simulink subsystem "Sensores"  (R2022b)
settings: Solver=VariableStepAuto  StartTime=0.0  StopTime=10.0  RelTol=1e-3
libraries: arduinolib x2
settings Model: Creator=mmgac  LastModifiedBy=mmgac

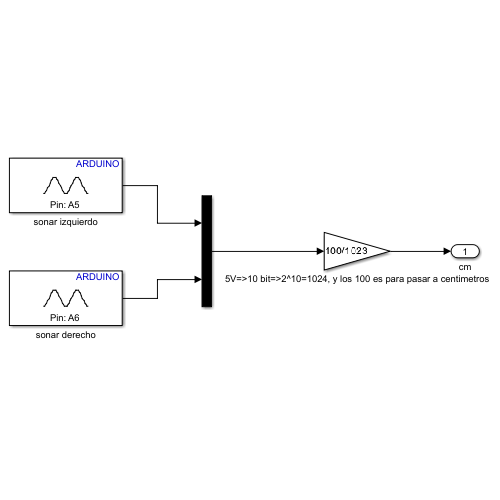
[thumbnail: Simulink's stored preview of the top-level diagram]
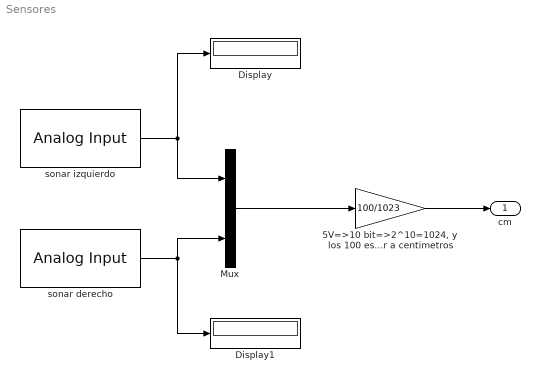
== system Sensores ==
  "5V=>10 bit=>2^10=1024, y los 100 es para pasar a centimetros" : Gain  Gain=100/1023
  Display : Display
  Display1 : Display
  Mux : Mux  Inputs=2
  sonar derecho : arduinolib/Analog Input  pinNumber=6  ReadResultsOnly=off  ConversionTriggerSource=Software  ExternalTriggerType=uint32( 0 )  OutputDataType=uint16  EnableConversionCompleteNotify=off  EnableOuputStatus=off  SampleTime=0.1  blockPlatform=arduino
  sonar izquierdo : arduinolib/Analog Input  pinNumber=5  ReadResultsOnly=off  ConversionTriggerSource=Software  ExternalTriggerType=uint32( 0 )  OutputDataType=uint16  EnableConversionCompleteNotify=off  EnableOuputStatus=off  SampleTime=0.1  blockPlatform=arduino
  cm : Outport
  wires:
  sonar izquierdo/1 -> Mux/1, Display/1
  sonar derecho/1 -> Mux/2, Display1/1
  Mux/1 -> "5V=>10 bit=>2^10=1024, y los 100 es para pasar a centimetros"/1
  "5V=>10 bit=>2^10=1024, y los 100 es para pasar a centimetros"/1 -> cm/1
